simulink model "stridac_3f"  (Simulink 8.0)
settings: Solver=ode1  StartTime=0.0  StopTime=0.5  FixedStep=1e-5  RelTol=1e-3
undefined symbols (not defined in the file): plecsedit
libraries: simulink x1
settings Model: Creator=kaskaj  LastModifiedBy=Kasi
settings DataIOCC: SignalLoggingSaveFormat=ModelDataLogs
settings DebuggingCC: FcnCallInpInsideContextMsg=UseLocalSettings
settings GRTTargetCC: CombineOutputUpdateFcns=off  GRTInterface=on

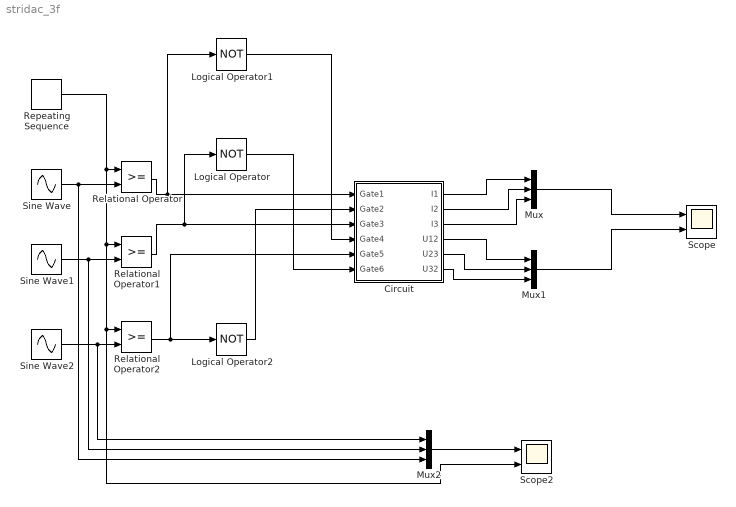
== system stridac_3f ==
  Circuit : Subsystem  LoadFcn=plecsedit('sl', 200);  InitFcn=plecsedit('sl', 214);  StartFcn=plecsedit('sl', 208);  StopFcn=plecsedit('sl', 209);  mask(PlecsCircuit){}
      mask init:
      | % PLACE CUSTOM INITIALIZATIONS ABOVE
      | % DO NOT REMOVE
      | plecsedit('sl', 215);
      | % DO NOT REMOVE
      settings: CopyFcn=plecsedit('sl', 203);  DeleteFcn=plecsedit('sl', 205);  UndoDeleteFcn=plecsedit('sl', 206);  PreSaveFcn=plecsedit('sl', 211);  PostSaveFcn=plecsedit('sl', 201);  NameChangeFcn=plecsedit('sl', 210);  DestroyFcn=plecsedit('sl', 207);  PreCopyFcn=plecsedit('sl', 216);  OpenFcn=plecsedit('sl', 202);  ErrorFcn=plerrorfcn
      mask Display: disp('PLECS\nCircuit')
  Logical Operator : Logic  Operator=NOT  AllPortsSameDT=off  OutDataTypeStr=boolean
  Logical Operator1 : Logic  Operator=NOT  AllPortsSameDT=off  OutDataTypeStr=boolean
  Logical Operator2 : Logic  Operator=NOT  AllPortsSameDT=off  OutDataTypeStr=boolean
  Mux : Mux  Inputs=3
  Mux1 : Mux  Inputs=3
  Mux2 : Mux  Inputs=3
  Relational Operator : RelationalOperator  OutDataTypeStr=boolean
  Relational Operator1 : RelationalOperator  OutDataTypeStr=boolean
  Relational Operator2 : RelationalOperator  OutDataTypeStr=boolean
  Repeating Sequence : simulink/Sources/Repeating Sequence  rep_seq_t=[0 0.5 1]/1000  rep_seq_y=[-1 1 -1]
  Scope : Scope  NumInputPorts=2
      settings: TimeRange=0.5  YMin=-700~-200  YMax=700~200
  Scope2 : Scope  NumInputPorts=2
      settings: YMin=-1~-5  YMax=1~5  SaveName=ScopeData2
  Sine Wave : Sin  Frequency=50  SampleTime=0
  Sine Wave1 : Sin  Frequency=50  Phase=(2*pi)/(3)  SampleTime=0
  Sine Wave2 : Sin  Frequency=50  Phase=(4*pi)/3  SampleTime=0
  wires:
  Mux2/1 -> Scope2/1
  Mux/1 -> Scope/1
  Mux1/1 -> Scope/2
  Circuit/1(I1) -> Mux/1
  Circuit/2(I2) -> Mux/2
  Circuit/3(I3) -> Mux/3
  Circuit/4(U12) -> Mux1/1
  Circuit/5(U23) -> Mux1/2
  Circuit/6(U32) -> Mux1/3
  Sine Wave/1 -> Mux2/3, Relational Operator/2
  Sine Wave1/1 -> Mux2/2, Relational Operator1/2
  Sine Wave2/1 -> Mux2/1, Relational Operator2/2
  Repeating Sequence/1 -> Scope2/2, Relational Operator2/1, Relational Operator1/1, Relational Operator/1
  Relational Operator/1 -> Logical Operator1/1, Circuit/1(Gate1)
  Relational Operator1/1 -> Logical Operator/1, Circuit/3(Gate3)
  Relational Operator2/1 -> Logical Operator2/1, Circuit/5(Gate5)
  Logical Operator2/1 -> Circuit/2(Gate2)
  Logical Operator1/1 -> Circuit/4(Gate4)
  Logical Operator/1 -> Circuit/6(Gate6)

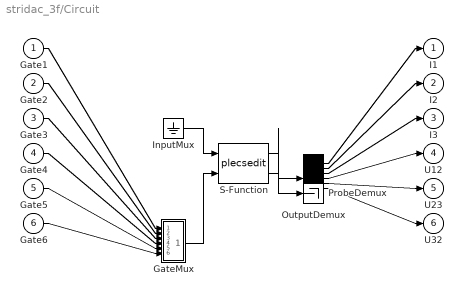
== system stridac_3f/Circuit ==
  Gate1 : Inport  PortDimensions=1
  Gate2 : Inport  Port=2  PortDimensions=1
  Gate3 : Inport  Port=3  PortDimensions=1
  Gate4 : Inport  Port=4  PortDimensions=1
  Gate5 : Inport  Port=5  PortDimensions=1
  Gate6 : Inport  Port=6  PortDimensions=1
  " GateMux " : Subsystem
      mask Display: disp('Mux')
  " InputMux " : Ground
  " OutputDemux " : Demux  Outputs=[ 1 1 1 1 1 1 ]
  " ProbeDemux " : Terminator
  " S-Function " : S-Function  FunctionName=plecsedit  EnableBusSupport=off
  I1 : Outport  PortDimensions=1
  I2 : Outport  Port=2  PortDimensions=1
  I3 : Outport  Port=3  PortDimensions=1
  U12 : Outport  Port=4  PortDimensions=1
  U23 : Outport  Port=5  PortDimensions=1
  U32 : Outport  Port=6  PortDimensions=1
  wires:
  " S-Function "/1 -> " OutputDemux "/1
  " InputMux "/1 -> " S-Function "/1
  " GateMux "/1(Out) -> " S-Function "/2
  " S-Function "/2 -> " ProbeDemux "/1
  Gate1/1 -> " GateMux "/1(In1)
  Gate2/1 -> " GateMux "/2(In2)
  Gate3/1 -> " GateMux "/3(In3)
  Gate4/1 -> " GateMux "/4(In4)
  Gate5/1 -> " GateMux "/5(In5)
  Gate6/1 -> " GateMux "/6(In6)
  " OutputDemux "/1 -> I1/1
  " OutputDemux "/2 -> I2/1
  " OutputDemux "/3 -> I3/1
  " OutputDemux "/4 -> U12/1
  " OutputDemux "/5 -> U23/1
  " OutputDemux "/6 -> U32/1

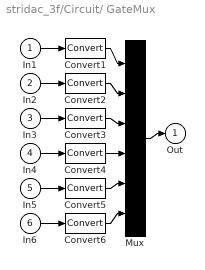
== system stridac_3f/Circuit/ GateMux  ==
  In1 : Inport
  In2 : Inport  Port=2
  In3 : Inport  Port=3
  In4 : Inport  Port=4
  In5 : Inport  Port=5
  In6 : Inport  Port=6
  Convert{1..6} (6 alike) : DataTypeConversion  SaturateOnIntegerOverflow=on  RndMeth=Zero
  Mux : Mux  Inputs=[ 1 1 1 1 1 1 ]
  Out : Outport
  wires:
  Mux/1 -> Out/1
  In1/1 -> Convert1/1
  In2/1 -> Convert2/1
  In3/1 -> Convert3/1
  In4/1 -> Convert4/1
  In5/1 -> Convert5/1
  In6/1 -> Convert6/1
  Convert1/1 -> Mux/1
  Convert2/1 -> Mux/2
  Convert3/1 -> Mux/3
  Convert4/1 -> Mux/4
  Convert5/1 -> Mux/5
  Convert6/1 -> Mux/6
